simulink model "State_Machine"  (R2021a)
settings: Solver=VariableStepAuto  StartTime=0.0  StopTime=10.0  RelTol=1e-3
settings Model: Creator=kbhar  LastModifiedBy=kbhar

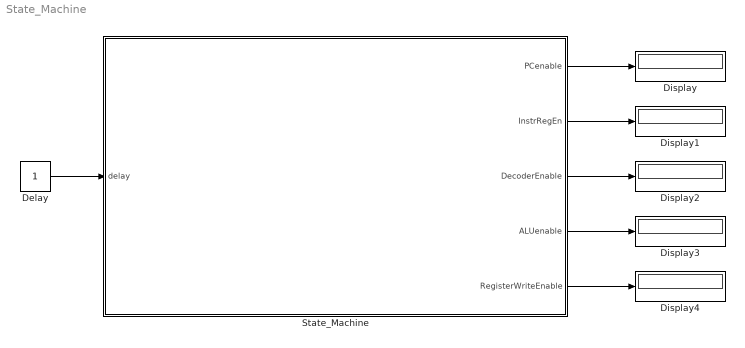
== system State_Machine ==
  Delay : Constant
  Display{,1..4} (5 alike) : Display
  State_Machine : Stateflow chart  TreatAsAtomicUnit=on
  wires:
  Delay/1 -> State_Machine/1(delay)
  State_Machine/4(ALUenable) -> Display3/1
  State_Machine/1(PCenable) -> Display/1
  State_Machine/3(DecoderEnable) -> Display2/1
  State_Machine/2(InstrRegEn) -> Display1/1
  State_Machine/5(RegisterWriteEnable) -> Display4/1

== stateflow chart State_Machine/State_Machine ==
  state start
    PCenable = 0; InstrRegEn = 0; DecoderEnable = 0; ALUenable = 0; RegisterWriteEnable = 0;
  state Fetch
    PCenable = 1; InstrRegEn = 1; DecoderEnable = 0; ALUenable = 0; RegisterWriteEnable = 0;
  state Decode
    PCenable = 0; InstrRegEn = 0; DecoderEnable = 1; ALUenable = 0; RegisterWriteEnable = 0;
  state Execute
    PCenable = 0; InstrRegEn = 0; DecoderEnable = 0; ALUenable = 1; RegisterWriteEnable = 0;
  state Writeback
    PCenable = 0; InstrRegEn = 0; DecoderEnable = 0; ALUenable = 0; RegisterWriteEnable = 1;
  (default) -> start
  start -> Fetch
  Writeback -> Fetch : [delay > 40]
  Fetch -> Decode : [delay > 10]
  Decode -> Execute : [delay > 20]
  Execute -> Writeback : [delay > 30]
  data: delay input; PCenable output; InstrRegEn output; DecoderEnable output; ALUenable output; RegisterWriteEnable output
